simulink model "GVCU_HIL"  (R2026a)
settings: Solver=ode3  StartTime=0  StopTime=2474  FixedStep=0.0002
model workspace (MAT data in the model file):
  CANoelibParameters : object (value not decoded)
values from neighbouring files (symbols this model uses):
  acc_pedal_data = pedal_data.accelerator_pedal_position_t0    [Vehicle_Simulink_init.m]
  acc_pedal_time = pedal_data.t0    [Vehicle_Simulink_init.m]
  brk_pedal_data = brake_pedal_data.shared_brakes_drvrBrkPedlPerc_t0    [Vehicle_Simulink_init.m]
  brk_pedal_time = brake_pedal_data.t0    [Vehicle_Simulink_init.m]
  cycle_len = zeros(1, num_cycles)    [Vehicle_Simulink_init.m]
  cycle_speed_matrix = zeros(max_cycle_len, num_cycles)    [Vehicle_Simulink_init.m]
  cycle_time_matrix = zeros(max_cycle_len, num_cycles)    [Vehicle_Simulink_init.m]
  veh_speed_data = speed_data.shared_dynamicsVso_vehVelLgt_t0    [Vehicle_Simulink_init.m]
  veh_speed_time = speed_data.t0    [Vehicle_Simulink_init.m]
undefined symbols (not defined in the file or in its folder): Active, AuxActive, bat, environment, FL_prs_voltage, FR_prs_voltage, pos, RL_prs_voltage, RR_prs_voltage, tir, veh, VGetRawValueFlag, Voltage, VT2816_1_Ch1, VT2816_1_Ch2, VT2816_1_Ch3, VT2816_1_Ch4, VT2816_3_Ch13, VT2816_3_Ch14, VT7101_1_Out2, VT7820_2_Channel1, VT7820_2_Channel2, VT7820_2_Channel3, VT7820_2_Channel4, VTS
libraries: canoelib x144, autolibsharedcoupling x21, autolibcoupling x9, autolibshared x5, simulink_extras x4, simulink x4, slpidlib x3, autolibshareddiff x3, autolibutils x1, autolibdatasheetbattery x1, autolibmappedmotor x1, sl_discontinuities x1
(part 6 of 9)

== system GVCU_HIL/Powertrain (EV)/EM ==
  note: recuperation
  TrqCmd : Inport
  EMSpd : Inport  Port=2
  Bus Creator : BusCreator  Inputs=3
  Constant : Constant
  Constant1 : Constant  Value=-1
  Datasheet Battery2 : autolibdatasheetbattery/Datasheet Battery  CapacityCtrl=Parameter  OutputVlt=Unfiltered  BattChargeMax=14.118  Em=[706.554, 720.834, 735.216, 742.356, 750.72, 765.714, 790.704, 810.798, 832.524, 855.372]  SOCEmBp=[0.1, 0.2, 0.3, 0.4, 0.5, 0.6, 0.7, 0.8, 0.9, 1]  RInt=[0.14, 0.12;0.14, 0.12;0.14, 0.12;0.14, 0.12;0.14, 0.12;0.14, 0.12;0.155, 0.135;0.16, 0.145;0.165, 0.155;0.175, 0.175]'  BattTempBp=|  SOCRintBp=[0.1, 0.2, 0.3, 0.4, 0.5, 0.6, 0.7, 0.8, 0.9, 1]  Ns=1  Np=1  BattCapInit=14.118*bat.SoC_init  Tc=1/1000  Vinit=4.221  RefBlkName='autolibdatasheetbattery/Datasheet Battery'
      | [318.15,
      | 333.15
      | ]
  Mapped Motor : autolibmappedmotor/Mapped Motor  w_Tmax_bp_ext=w_Tmax_bp  Tmax_w_V_ext=Tmax_w_V  w_Tmin_bp_ext=w_Tmin_bp  Tmin_w_V_ext=Tmin_w_V  port_config=Speed  param_by=Tabulated torque-speed envelope  w_t=vEM  T_t=MEM  torque_max=.1  power_max=30  SpreadsheetTqLimitsFileName=MotorCalibrationImportData.xlsx  Tmax_w_V=[0.09 0.09 0.09;0.08 0.08 0.08;0.07 0.07 0.07;0 0 0]  w_Tmax_bp=[ 0 375 750 800 ]  V_Tmax_bp=[500 750 900]  Tmin_w_V=[-0.09 -0.09 -0.09;-0.08 -0.08 -0.08;-0.07 -0.07 -0.07;0 0 0]  w_Tmin_bp=[ 0 375 750 800 ]  V_Tmin_bp=[500 750 900]  Tc=0.02  param_loss=Tabulated loss data  SpreadsheetLossFileName=MotorCalibrationImportData.xlsx  SpreadsheetEffFileName=MotorCalibrationImportData.xlsx  eff=100  w_eff=375  T_eff=0.08  Piron=0  Pbase=0  w_eff_bp=eff_EM_speed  T_eff_bp=eff_EM_torque  Temp_eff_bp=[233.15 293.15 373.15]  V_eff_bp=[500 700 900]  losses_table=eff_EM_loss'  losses_table_3d=cat(3,[1.49 1.67 2.21 3.10; 0.42 0.69 1.14 2.03; 0.06 0.24 0.78 1.68; 0.42 0.69 1.14 2.03; 1.49 1.67 2.21 3.10],[1.49 1.67 2.21 3.10; 0.42 0.69 1.14 2.03; 0.06 0.24 0.78 1.68; 0.42 0.69 1.14 2.03; 1.49 1.67 2.21 3.10],[1.49 1.67 2.21 3.10; 0.42 0.69 1.14 2.03; 0.06 0.24 0.78 1.68; 0.42 0.69 1.14 2.03; 1.49 1.67 2.21 3.10])  losses_table_4d=cat(4,cat(3,[1.5645 0.441 0.063 0.441 1.5645;1.7535 0.7245 0.252 0.7245 1.7535;2.3205 1.197 0.819 1.197 2.3205;3.255 2.1315 1.764 2.1315 3.255],[1.5645 0.441 0.063 0.441 1.5645;1.7535 0.7245 0.252 0.7245 1.7535;2.3205 1.197 0.819 1.197 2.3205;3.255 2.1315 1.764 2.1315 3.255],[1.5645 0.441 0.063 0.441 1.5645;1.7535 0.7245 0.252 0.7245 1.7535;2.3205 1.197 0.819 1.197 2.3205;3.255 2.1315 1.764 2.1315 3.255]),cat(3,[1.49 0.42 0.06 0.42 1.49;1.67 0.69 0.24 0.69 1.67;2.21 1.14 0.78 1.14 2.21;3.1 2.03 1.68 2.03 3.1],[1.49 0.42 0.06 0.42 1.49;1.67 0.69 0.24 0.69 1.67;2.21 1.14 0.78 1.14 2.21;3.1 2.03 1.68 2.03 3.1],[1.49 0.42 0.06 0.42 1.49;1.67 0.69 0.24 0.69 1.67;2.21 1.14 0.78 1.14 2.21;3.1 2.03 1.68 2.03 3.1]),cat(3,[1.5347 0.4326 0.0618 0.4326 1.5347;1.7201 0.7107 0.2472 0.7107 1.7201;2.2763 1.1742 0.8034 1.1742 2.2763;3.193 2.0909 1.7304 2.0909 3.193],[1.5347 0.4326 0.0618 0.4326 1.5347;1.7201 0.7107 0.2472 0.7107 1.7201;2.2763 1.1742 0.8034 1.1742 2.2763;3.193 2.0909 1.7304 2.0909 3.193],[1.5347 0.4326 0.0618 0.4326 1.5347;1.7201 0.7107 0.2472 0.7107 1.7201;2.2763 1.1742 0.8034 1.1742 2.2763;3.193 2.0909 1.7304 2.0909 3.193]))  efficiency_table=[95 95 95 95; 95 95 95 95; 95 95 95 95; 95 95 95 95; 95 95 95 95]  efficiency_table_3d=cat(3,[95 95 95 95; 95 95 95 95; 95 95 95 95; 95 95 95 95; 95 95 95 95],[95 95 95 95; 95 95 95 95; 95 95 95 95; 95 95 95 95; 95 95 95 95],[95 95 95 95; 95 95 95 95; 95 95 95 95; 95 95 95 95; 95 95 95 95])  efficiency_table_4d=cat(4,cat(3,90*ones(5,4)',90*ones(5,4)',90*ones(5,4)'),cat(3,95*ones(5,4)',95*ones(5,4)',95*ones(5,4)'),cat(3,92*ones(5,4)',92*ones(5,4)',92*ones(5,4)'))  J=5e-6  b=1e-5  omega_o=0  T_t_extended=[591.1765761 597.3209021 603.5893235 609.9750859 616.4522479 623.0217147 629.6859649 636.4772464 643.4544242 650.5325557 657.7142528 665.0004238 672.3918517 679.8891731 687.4928554 695.2382707 703.2239794 711.3175267 719.5183987 727.8257293 736.2382506 744.7548459 753.4914197 762.3651559 771.3359703 780.40539 789.5706985 798.8284396 808.4176374 818.1172796 827.8944537 837.7411079 847.6338253 857.4187059 867.2137586 877.0119255 886.7904649 896.5231126 906.1796142 915.3256846 924.6270531 933.8736555 942.8047497 951.8719913 960.6156155 968.6277666 976.0298627 982.43675 988.6022535 994.0259096 997.4001374 999.7922394 1000.534965 1000.5472 1000.5472 1000.5472 1000.5472 1000.5472 1000.5472 1000.5472 1000.5472 1000.5472 1000.5472 1000.5472 1000.5472 1000.5472 1000.5472 1000.5472 1000.5472 1000.5472 1000.5472 1000.5472 1000.5472 1000.5472 1000.5472 1000.5472 1000.5472 1000.5472 1000.5472 1000.5472 1000.5472 1000.5472 1000.5472 1000.5472 1000.5472 1000.5472 1000.5472 1000.5472 1000.5472 1000.5472 1000.5472 1000.5472 1000.5472 1000.5472 1000.5472 1000.5472 1000.5472 1000.5472 1000.5472 1000.5472 1000.5472 1000.5472 1000.5472 1000.5472 1000.5472 1000.5472 1000.5472 1000.5472 1000.5472 1000.5472 1000.5472 1000.5472 1000.5472 1000.5472 1000.5472 1000.5472 1000.5472 1000.5472 1000.5472 1000.5472 1000.5472 1000.5472 1000.5472 1000.5472 1000.5472 1000.5472 1000.5472 1000.5472 1000.5472 1000.5472 1000.5472 1000.5472 1000.5472 1000.5472 1000.5472 1000.5472 1000.5472 1000.5472 1000.5472 1000.5472 1000.5472 1000.5472 1000.5472 1000.5472 1000.5472 1000.5472 1000.5472 1000.5472 1000.534965 999.7922394 997.4001374 994.0259096 988.6022535 982.43675 976.0298627 968.6277666 960.6156155 951.8719913 942.8047497 933.8736555 924.6270531 915.3256846 906.1796142 896.5231126 886.7904649 877.0119255 867.2137586 857.4187059 847.6338253 837.7411079 827.8944537 818.1172796 808.4176374 798.8284396 789.5706985 780.40539 771.3359703 762.3651559 753.4914197 744.7548459 736.2382506 727.8257293 719.5183987 711.3175267 703.2239794 695.2382707 687.4928554 679.8891731 672.3918517 665.0004238 657.7142528 650.5325557 643.4544242 636.4772464 629.6859649 623.0217147 616.4522479 609.9750859 603.5893235 597.3209021 591.1765761]  w_t_extended=[-1047.197551 -1036.725576 -1026.2536 -1015.781625 -1005.309649 -994.8376736 -984.3656981 -973.8937226 -963.4217471 -952.9497716 -942.4777961 -932.0058206 -921.5338451 -911.0618695 -900.589894 -890.1179185 -879.645943 -869.1739675 -858.701992 -848.2300165 -837.758041 -827.2860654 -816.8140899 -806.3421144 -795.8701389 -785.3981634 -774.9261879 -764.4542124 -753.9822369 -743.5102613 -733.0382858 -722.5663103 -712.0943348 -701.6223593 -691.1503838 -680.6784083 -670.2064328 -659.7344573 -649.2624817 -638.7905062 -628.3185307 -617.8465552 -607.3745797 -596.9026042 -586.4306287 -575.9586532 -565.4866776 -555.0147021 -544.5427266 -534.0707511 -523.5987756 -513.1268001 -502.6548246 -492.1828491 -481.7108736 -471.238898 -460.7669225 -450.294947 -439.8229715 -429.350996 -418.8790205 -408.407045 -397.9350695 -387.4630939 -376.9911184 -366.5191429 -356.0471674 -345.5751919 -335.1032164 -324.6312409 -314.1592654 -303.6872898 -293.2153143 -282.7433388 -272.2713633 -261.7993878 -251.3274123 -240.8554368 -230.3834613 -219.9114858 -209.4395102 -198.9675347 -188.4955592 -178.0235837 -167.5516082 -157.0796327 -146.6076572 -136.1356817 -125.6637061 -115.1917306 -104.7197551 -94.24777961 -83.7758041 -73.30382858 -62.83185307 -52.35987756 -41.88790205 -31.41592654 -20.94395102 -10.47197551 0 10.47197551 20.94395102 31.41592654 41.88790205 52.35987756 62.83185307 73.30382858 83.7758041 94.24777961 104.7197551 115.1917306 125.6637061 136.1356817 146.6076572 157.0796327 167.5516082 178.0235837 188.4955592 198.9675347 209.4395102 219.9114858 230.3834613 240.8554368 251.3274123 261.7993878 272.2713633 282.7433388 293.2153143 303.6872898 314.1592654 324.6312409 335.1032164 345.5751919 356.0471674 366.5191429 376.9911184 387.4630939 397.9350695 408.407045 418.8790205 429.350996 439.8229715 450.294947 460.7669225 471.238898 481.7108736 492.1828491 502.6548246 513.1268001 523.5987756 534.0707511 544.5427266 555.0147021 565.4866776 575.9586532 586.4306287 596.9026042 607.3745797 617.8465552 628.3185307 638.7905062 649.2624817 659.7344573 670.2064328 680.6784083 691.1503838 701.6223593 712.0943348 722.5663103 733.0382858 743.5102613 753.9822369 764.4542124 774.9261879 785.3981634 795.8701389 806.3421144 816.8140899 827.2860654 837.758041 848.2300165 858.701992 869.1739675 879.645943 890.1179185 900.589894 911.0618695 921.5338451 932.0058206 942.4777961 952.9497716 963.4217471 973.8937226 984.3656981 994.8376736 1005.309649 1015.781625 1026.2536 1036.725576 1047.197551]  KLossIron=0  KLossCopper=0  x_w_eff_vec=[-1151.91730631626 -1099.55742875643 -1047.1975511966 -994.837673636768 -942.477796076938 -890.117918517108 -837.758040957278 -785.398163397448 -733.038285837618 -680.678408277789 -628.318530717959 -575.958653158129 -523.598775598299 -471.238898038469 -418.879020478639 -366.519142918809 -314.159265358979 -261.799387799149 -209.43951023932 -157.07963267949 -104.71975511966 -52.3598775598299 0 52.3598775598299 104.71975511966 157.07963267949 209.43951023932 261.799387799149 314.159265358979 366.519142918809 418.879020478639 471.238898038469 523.598775598299 575.958653158129 628.318530717959 680.678408277789 733.038285837618 785.398163397448 837.758040957278 890.117918517108 942.477796076938 994.837673636768 1047.1975511966 1099.55742875643 1151.91730631626]  x_T_eff_vec=[-1100 -1000 -900 -800 -700 -600 -500 -400 -300 -200 -100 0 100 200 300 400 500 600 700 800 900 1000 1100]  x_tmp_eff_vec=[-0.09 -0.06 -0.03 0 0.03 0.06 0.09]  x_V_eff_vec=[500 700 900]  x_losses_mat=[216963.75801 216996.227265 206067.578848888 197642.105612969 153300.977107873 108080.0572 72647.49686 49091.12876 32858.35954 22129.50585 16054.65961 13895.5575 16054.65961 22129.50585 32858.35954 49091.12876 72647.49686 108080.0572 153300.977107873 197642.105612969 206067.578848888 216996.227265 216963.75801;231488.890349682 223059.669245745 204039.410989428 184347.436290099 134715.207987873 87903.07434 59579.3291 40088.01049 26456.98289 17357.92244 12141.80753 10371.65043 12141.80753 17357.92244 26456.98289 40088.01049 59579.3291 87903.07434 134715.207987873 184347.436290099 204039.410989428 223059.669245745 231488.890349682;189437.61777 184243.717645 168828.860886349 149567.396061484 106341.0793 71543.39502 48728.82856 32631.17131 21200.63415 13523.21842 9082.511039 7599.257015 9082.511039 13523.21842 21200.63415 32631.17131 48728.82856 71543.39502 106341.0793 149567.396061484 168828.860886349 184243.717645 189437.61777;192935.210247969 180472.732852227 158159.379341563 128824.526141484 85033.49473 58268.77005 39819.67343 26520.36346 16954.07308 10512.49572 6795.723221 5551.699791 6795.723221 10512.49572 16954.07308 26520.36346 39819.67343 58268.77005 85033.49473 128824.526141484 158159.379341563 180472.732852227 192935.210247969;155580.94976 146657.635255 128253.525153809 99653.02374 68484.12552 47553.88198 32618.55146 21582.78411 13649.90656 8283.638962 5179.539664 4137.799792 5179.539664 8283.638962 13649.90656 21582.78411 32618.55146 47553.88198 68484.12552 99653.02374 128253.525153809 146657.635255 155580.94976;129871.92913 122034.11486 105085.58551254 79050.02512 55595.93478 39058.96664 26875.37628 17810.73423 11257.11835 6780.923192 4207.530813 3337.757479 4207.530813 6780.923192 11257.11835 17810.73423 26875.37628 39058.96664 55595.93478 79050.02512 105085.58551254 122034.11486 129871.92913;121153.617618809 109771.61748004 89648.9827825395 64650.328115 45845.19165 32428.08909 22502.00533 15114.9243 9718.777596 5996.518981 3863.3287 3140.213628 3863.3287 5996.518981 9718.777596 15114.9243 22502.00533 32428.08909 45845.19165 64650.328115 89648.9827825395 109771.61748004 121153.617618809;102556.24812 91278.85608 71630.91 52385.27894 38216.08162 27475.52514 19481.57898 13474.37309 8882.641372 5572.115215 3606.515506 2926.128354 3606.515506 5572.115215 8882.641372 13474.37309 19481.57898 27475.52514 38216.08162 52385.27894 71630.91 91278.85608 102556.24812;92639.38668 78466.74469 58974.42114 44130.45585 32866.66791 24279.62179 17574.57444 12226.59488 8087.099664 5111.496599 3338.107135 2693.28051 3338.107135 5111.496599 8087.099664 12226.59488 17574.57444 24279.62179 32866.66791 44130.45585 58974.42114 78466.74469 92639.38668;79967.9231 65252.31828 50217.87648 38582.89904 29358.82442 21876.86476 15843.69216 11050.03907 7345.279935 4716.81461 3049.949208 2447.800925 3049.949208 4716.81461 7345.279935 11050.03907 15843.69216 21876.86476 29358.82442 38582.89904 50217.87648 65252.31828 79967.9231;71978.46712 56942.67707 44620.193540345 34536.29737 26359.17892 19662.58912 14256.71192 9978.264251 6676.859148 4212.93021 2749.898985 2203.255002 2749.898985 4212.93021 6676.859148 9978.264251 14256.71192 19662.58912 26359.17892 34536.29737 44620.193540345 56942.67707 71978.46712;64307.84812 50926.57919 39881.7876028249 30906.36917 23642.38009 17643.48449 12827.89413 8955.839244 5908.871417 3769.457125 2456.82187 1959.642739 2456.82187 3769.457125 5908.871417 8955.839244 12827.89413 17643.48449 23642.38009 30906.36917 39881.7876028249 50926.57919 64307.84812;57412.00559 45490.46778 35625.4624361057 27664.12726 21175.22168 15830.68178 11431.8958 7924.881587 5262.677959 3349.859461 2170.073056 1716.964138 2170.073056 3349.859461 5262.677959 7924.881587 11431.8958 15830.68178 21175.22168 27664.12726 35625.4624361057 45490.46778 57412.00559;51224.02114 40607.66616 31797.2898800987 24744.95924 18926.39057 14056.32423 10116.63964 7040.932836 4665.120485 2950.41808 1889.056344 1475.219198 1889.056344 2950.41808 4665.120485 7040.932836 ...(+8994 chars)]  x_losses_mat_3d=[37.8947368421052 25.2631578947368 12.6315789473684 0 12 24 36;18.9473684210526 12.6315789473684 6.3157894736842 0 5.99999999999999 12 18;0 0 0 0 0 0 0;18 12 5.99999999999999 0 6.3157894736842 12.6315789473684 18.9473684210526;36 24 12 0 12.6315789473684 25.2631578947368 37.8947368421052]  x_losses_mat_4d=cat(4,cat(3,[1.5645 0.441 0.063 0.441 1.5645;1.7535 0.7245 0.252 0.7245 1.7535;2.3205 1.197 0.819 1.197 2.3205;3.255 2.1315 1.764 2.1315 3.255],[1.5645 0.441 0.063 0.441 1.5645;1.7535 0.7245 0.252 0.7245 1.7535;2.3205 1.197 0.819 1.197 2.3205;3.255 2.1315 1.764 2.1315 3.255],[1.5645 0.441 0.063 0.441 1.5645;1.7535 0.7245 0.252 0.7245 1.7535;2.3205 1.197 0.819 1.197 2.3205;3.255 2.1315 1.764 2.1315 3.255]),cat(3,[1.49 0.42 0.06 0.42 1.49;1.67 0.69 0.24 0.69 1.67;2.21 1.14 0.78 1.14 2.21;3.1 2.03 1.68 2.03 3.1],[1.49 0.42 0.06 0.42 1.49;1.67 0.69 0.24 0.69 1.67;2.21 1.14 0.78 1.14 2.21;3.1 2.03 1.68 2.03 3.1],[1.49 0.42 0.06 0.42 1.49;1.67 0.69 0.24 0.69 1.67;2.21 1.14 0.78 1.14 2.21;3.1 2.03 1.68 2.03 3.1]),cat(3,[1.5347 0.4326 0.0618 0.4326 1.5347;1.7201 0.7107 0.2472 0.7107 1.7201;2.2763 1.1742 0.8034 1.1742 2.2763;3.193 2.0909 1.7304 2.0909 3.193],[1.5347 0.4326 0.0618 0.4326 1.5347;1.7201 0.7107 0.2472 0.7107 1.7201;2.2763 1.1742 0.8034 1.1742 2.2763;3.193 2.0909 1.7304 2.0909 3.193],[1.5347 0.4326 0.0618 0.4326 1.5347;1.7201 0.7107 0.2472 0.7107 1.7201;2.2763 1.1742 0.8034 1.1742 2.2763;3.193 2.0909 1.7304 2.0909 3.193]))  CalLossMapData={}  CalLossWithTempMapData={}  aMode=1  RefBlkName='autolibmappedmotor/Mapped Motor'
      settings: LibrarySourceBlock=autolibemachines/Mapped Motor
  Product : Product
  Product1 : Product
  Switch : Switch  SaturateOnIntegerOverflow=off  InputSameDT=off
  System Variable Output : canoelib/CANoe I//O/System Variable Output  Commented=on  nsName=Checker_Simulink  sysVarName=Test_param  arrayIndex=-1  rawValue=Default  dataType=Default  dataTypeDB=int32  hasEncoding=off  dataTypeCANoe=Get from CANoe
      settings: AttributesFormatString=%<nsName>::%<sysVarName>  SourceProductName=Vector CANoe
  Temperature1 : Constant  Value=320
  Terminator : Terminator
  Transfer Fcn : TransferFcn  Denominator=[0.001 1]
  Info : Outport
  EMTrq : Outport  Port=2  VectorParamsAs1DForOutWhenUnconnected=off
  tag scope: BatteryCurrent=global, BatteryVoltage=global
  wires:
  Mapped Motor/2 -> Transfer Fcn/1
  Transfer Fcn/1 -> Datasheet Battery2/1, [BatteryCurrent]
  Datasheet Battery2/1 -> [Battery]  "Battery"
  [EMSpd] -> Bus Creator/1  "EMSpd"
  [Battery] -> Bus Creator/3  "Battery"
  Datasheet Battery2/2 -> Mapped Motor/1, [BatteryVoltage]  "New"
  Temperature1/1 -> Datasheet Battery2/2
  Bus Creator/1 -> Info/1
  EMSpd/1 -> Mapped Motor/2, [EMSpd]  "EMSpd"
  Product1/1 -> EMTrq/1, Bus Creator/2  "EMTrq"
  Mapped Motor/1 -> Terminator/1
  Constant/1 -> Switch/1
  Constant1/1 -> Switch/3
  Switch/1 -> Product/2, System Variable Output/1, Product1/2  "1 or -1"
  Product/1 -> Mapped Motor/3
  Mapped Motor/3 -> Product1/1  "EMTrq"
  TrqCmd/1 -> Switch/2, Product/1  "TrqCmd"

== system GVCU_HIL/Powertrain (EV)/FWD_ELEC_Powertrain ==
  EMTrq : Inport
  Veh : Inport  Port=2
  Bus Selector : BusSelector  OutputSignals=Wheels.Omega
  Constant2 : Constant  Value=0
  Constant3 : Constant  Value=0
  Demux : Demux
  FL : autolibsharedcoupling/Torsional Compliance  port_config=Simulink  extInfo=off  k=5e4  b=4e2  theta_o=0  domega_o=0  omega_c=3000  blkID=0  aMode=1
  FL_Clutch : autolibcoupling/Disc Clutch  port_config=Simulink  Reff=.091/2  Ndisk=9  Aeff=0.006283185  Peng=320000  Jin=.1  Jout=.1  muk=.088  mus=.089  bin=.001  bout=.001  win_o=pos.xdot_0/veh.TyreLoadedRadius_F  wout_o=pos.xdot_0/veh.TyreLoadedRadius_F  tauC=1  InitiallyLocked=off  maxAbsSpd=3000  blkID=1
  FR : autolibsharedcoupling/Torsional Compliance  port_config=Simulink  extInfo=off  k=5e4  b=4e2  theta_o=0  domega_o=0  omega_c=3000  blkID=0  aMode=1
  FR_Clutch : autolibcoupling/Disc Clutch  port_config=Simulink  Reff=.091/2  Ndisk=9  Aeff=0.006283185  Peng=320000  Jin=.1  Jout=.1  muk=.088  mus=.089  bin=.001  bout=.001  win_o=pos.xdot_0/veh.TyreLoadedRadius_F  wout_o=pos.xdot_0/veh.TyreLoadedRadius_F  tauC=.01  InitiallyLocked=off  maxAbsSpd=3000  blkID=1
  From1 : From  Commented=on  GotoTag=FR_prs  TagVisibility=global
  Gain : Gain  Gain=1/2.71
  Gain1 : Gain  Gain=1/2.71
  Gain2 : Gain  Gain=30/pi
  Mux1 : Mux
  Rotational Inertia : autolibsharedcoupling/Rotational Inertia  port_config=Simulink  extInfo=off  externJ=off  J=.1  b=.001  omega_o=0  blkID=0  aMode=1
      settings: LibrarySourceBlock=autolibcoupling/Rotational Inertia
  Split Torsional Compliance : autolibsharedcoupling/Split Torsional Compliance  port_config=Simulink  cplrMode=Shaft split  extInfo=off  k1=5e4  b1=4e2  omega1_c=1000  theta1_o=0  domega1_o=0  k2=5e4  b2=4e2  omega2_c=1000  theta2_o=0  domega2_o=0  blkID=0  aMode=1
      settings: LibrarySourceBlock=autolibcoupling/Split Torsional Compliance
  Terminator{,1..3} (4 alike) : Terminator
  EM_Spd : Outport
  Axl_Trq1 : Outport  Port=2
  tag scope: Axl_front_Spd=global, Split_tors_FL=global, Split_tors_FR=global
  wires:
  Constant3/1 -> Mux1/4
  Constant2/1 -> Mux1/3
  Mux1/1 -> Axl_Trq1/1
  FR/2 -> Mux1/2  "T_FR"
  FL/2 -> Mux1/1  "T_FL"
  EMTrq/1 -> Rotational Inertia/1
  Split Torsional Compliance/1 -> Gain1/1
  Demux/1 -> FL/2
  Split Torsional Compliance/3 -> [Split_tors_FR], FR_Clutch/2  "Front_right_clutch"
  FL_Clutch/1 -> Terminator3/1
  [FL_prs] -> FR_Clutch/1, FL_Clutch/1
  Veh/1 -> Bus Selector/1
  FR_Clutch/2 -> Split Torsional Compliance/3
  FR/1 -> FR_Clutch/3
  Split Torsional Compliance/2 -> [Split_tors_FL], FL_Clutch/2  "Front_left_clutch"
  Rotational Inertia/1 -> EM_Spd/1, Gain/1
  Gain/1 -> Gain2/1, Split Torsional Compliance/1
  Bus Selector/1 -> Demux/1  "<Omega>"
  FR_Clutch/3 -> FR/1
  Demux/4 -> Terminator1/1
  FR_Clutch/1 -> Terminator2/1
  FL_Clutch/2 -> Split Torsional Compliance/2
  Demux/2 -> FR/2
  Demux/3 -> Terminator/1
  FL_Clutch/3 -> FL/1
  FL/1 -> FL_Clutch/3
  Gain1/1 -> Rotational Inertia/2
  Gain2/1 -> [Axl_front_Spd]  "rpm"

== system GVCU_HIL/Powertrain (EV)/FWD_ELEC_Powertrain_sorted ==
  note: Front Bevel Ration
  EMTrq : Inport
  Veh : Inport  Port=2
  Bus Selector : BusSelector  OutputSignals=Wheels.Omega
  Constant2 : Constant  Value=0
  Constant3 : Constant  Value=0
  Demux : Demux
  FL : autolibsharedcoupling/Torsional Compliance  port_config=Simulink  extInfo=off  k=5e4  b=4e2  theta_o=0  domega_o=0  omega_c=3000  blkID=0  aMode=1
  FL_Clutch : autolibcoupling/Disc Clutch  port_config=Simulink  Reff=.091/2  Ndisk=9  Aeff=0.006283185  Peng=110000  Jin=.1  Jout=.1  muk=.088  mus=.089  bin=.001  bout=.001  win_o=pos.xdot_0/veh.TyreLoadedRadius_F  wout_o=pos.xdot_0/veh.TyreLoadedRadius_F  tauC=1  InitiallyLocked=off  maxAbsSpd=3000  blkID=1
  FR : autolibsharedcoupling/Torsional Compliance  port_config=Simulink  extInfo=off  k=5e4  b=4e2  theta_o=0  domega_o=0  omega_c=3000  blkID=0  aMode=1
  FR_Clutch : autolibcoupling/Disc Clutch  port_config=Simulink  Reff=.091/2  Ndisk=9  Aeff=0.006283185  Peng=110000  Jin=.1  Jout=.1  muk=.088  mus=.089  bin=.001  bout=.001  win_o=pos.xdot_0/veh.TyreLoadedRadius_F  wout_o=pos.xdot_0/veh.TyreLoadedRadius_F  tauC=.01  InitiallyLocked=off  maxAbsSpd=3000  blkID=1
  Gain : Gain  Gain=1/2.71
  Gain1 : Gain  Gain=1/2.71
  Gain2 : Gain  Gain=30/pi
  Mux1 : Mux
  Rotational Inertia : autolibsharedcoupling/Rotational Inertia  port_config=Simulink  extInfo=off  externJ=off  J=.1  b=.001  omega_o=0  blkID=0  aMode=1
      settings: LibrarySourceBlock=autolibcoupling/Rotational Inertia
  Split Torsional Compliance : autolibsharedcoupling/Split Torsional Compliance  port_config=Simulink  cplrMode=Shaft split  extInfo=off  k1=5e4  b1=4e2  omega1_c=1000  theta1_o=0  domega1_o=0  k2=5e4  b2=4e2  omega2_c=1000  theta2_o=0  domega2_o=0  blkID=0  aMode=1
      settings: LibrarySourceBlock=autolibcoupling/Split Torsional Compliance
  Terminator{,1..3} (4 alike) : Terminator
  EM_Spd : Outport
  Axl_Trq1 : Outport  Port=2
  tag scope: Axl_front_Spd=global, Split_tors_FL=global, Split_tors_FR=global, T_FL=global, T_FR=global
  wires:
  Constant3/1 -> Mux1/4
  Constant2/1 -> Mux1/3
  Mux1/1 -> Axl_Trq1/1
  FR/2 -> [T_FR]  "T_FR"
  FL/2 -> [T_FL]  "T_FL"
  EMTrq/1 -> Rotational Inertia/1
  Split Torsional Compliance/1 -> Gain1/1
  Demux/1 -> FL/2
  Split Torsional Compliance/2 -> [Split_tors_FR], FR_Clutch/2  "Front_right_clutch"
  FL_Clutch/1 -> Terminator3/1
  [FR_prs] -> FR_Clutch/1
  Veh/1 -> Bus Selector/1
  FR_Clutch/2 -> Split Torsional Compliance/2
  FR/1 -> FR_Clutch/3
  Split Torsional Compliance/3 -> [Split_tors_FL], FL_Clutch/2  "Front_left_clutch"
  Rotational Inertia/1 -> EM_Spd/1, Gain/1
  Gain/1 -> Gain2/1, Split Torsional Compliance/1
  Bus Selector/1 -> Demux/1  "<Omega>"
  FR_Clutch/3 -> FR/1
  Demux/4 -> Terminator1/1
  FR_Clutch/1 -> Terminator2/1
  FL_Clutch/2 -> Split Torsional Compliance/3
  Demux/2 -> FR/2
  Demux/3 -> Terminator/1
  FL_Clutch/3 -> FL/1
  FL/1 -> FL_Clutch/3
  Gain1/1 -> Rotational Inertia/2
  Gain2/1 -> [Axl_front_Spd]  "rpm"
  [T_FR] -> Mux1/2
  [T_FL] -> Mux1/1
  [FL_prs] -> FL_Clutch/1

== system GVCU_HIL/Powertrain (EV)/PID Speed Controller ==
  note: feed forward value
  speed_feedback : Inport
  trq_lim : Inport  Port=2
  speed_req : Inport  Port=3
  trq_req : Inport  Port=4
  reset : Inport  Port=5
  Add : Sum
  Add1 : Sum
  Clock : Clock
  Constant : Constant  Commented=on  Value=0
  Gain : Gain  Gain=-1
  MATLAB Function : MATLAB Function  TreatAsAtomicUnit=on
  PID Controller1 : slpidlib/PID Controller  Controller=PI  Form=Parallel  TimeDomain=Discrete-time  UseExternalTs=off  SampleTime=0.0004  IntegratorMethod=Trapezoidal  FilterMethod=Forward Euler  ControllerParametersSource=internal  P=0.78  I=0.01  UseKiTs=off  D=0  UseExternalDerivativeSource=off  N=100  UseFilter=on  TunerSelectOption=Transfer Function Based (PID Tuner App)  InitialConditionSource=internal  InitialConditionForIntegrator=0  InitialConditionForFilter=0  DifferentiatorICPrevScaledInput=0  ExternalReset=level  TrackingMode=off  Kt=1  LimitOutput=on  SatLimitsSource=internal  UpperSaturationLimit=1000  LowerSaturationLimit=-1000  LinearizeAsGain=on  AntiWindupMode=back-calculation  Kb=0.005  LimitIntegrator=on  UpperIntegratorSaturationLimit=inf  LowerIntegratorSaturationLimit=-inf  POutMin=[]  POutMax=[]  IOutMin=[]  IOutMax=[]  DOutMin=[]  DOutMax=[]  NOutMin=[]  NOutMax=[]  SumOutMin=[]  SumOutMax=[]  SaturationOutMin=[]  SaturationOutMax=[]  PParamMin=[]  PParamMax=[]  IParamMin=[]  IParamMax=[]  DParamMin=[]  DParamMax=[]  NParamMin=[]  NParamMax=[]  KbParamMin=[]  KbParamMax=[]  KtParamMin=[]  KtParamMax=[]  KbOutMin=[]  KbOutMax=[]  KtOutMin=[]  KtOutMax=[]  IntegratorOutMin=[]  IntegratorOutMax=[]  FilterOutMin=[]  FilterOutMax=[]  SumI1OutMin=[]  SumI1OutMax=[]  SumI2OutMin=[]  SumI2OutMax=[]  SumI3OutMin=[]  SumI3OutMax=[]  SumI4OutMin=[]  SumI4OutMax=[]  SumDOutMin=[]  SumDOutMax=[]  DifferentiatorOutMin=[]  DifferentiatorOutMax=[]  FilterDiffOutCoefMin=[]  FilterDiffOutCoefMax=[]  ReciprocalOutMin=[]  ReciprocalOutMax=[]  SumDenOutMin=[]  SumDenOutMax=[]  SumNumOutMin=[]  SumNumOutMax=[]  DivideOutMin=[]  DivideOutMax=[]  UdiffTsProdOutMin=[]  UdiffTsProdOutMax=[]  NTsProdOutMin=[]  NTsProdOutMax=[]  UintegralTsProdOutMin=[]  UintegralTsProdOutMax=[]  UngainTsProdOutMin=[]  UngainTsProdOutMax=[]  ClampingZeroOutDataTypeStr=Inherit: Inherit via back propagation  ClampingZeroOutMin=[]  ClampingZeroOutMax=[]  FilterDenConstantOutDataTypeStr=Inherit: Inherit via back propagation  FilterDenConstantOutMin=[]  FilterDenConstantOutMax=[]  PCopyOutDataTypeStr=Inherit: Inherit via back propagation  PCopyOutMin=[]  PCopyOutMax=[]  NCopyOutDataTypeStr=Inherit: Inherit via back propagation  NCopyOutMin=[]  NCopyOutMax=[]  IntegratorContinuousStateAttributes=''  IntegratorStateMustResolveToSignalObject=off  IntegratorRTWStateStorageClass=Auto  FilterContinuousStateAttributes=''  FilterStateMustResolveToSignalObject=off  FilterRTWStateStorageClass=Auto  ParallelPVariant=InternalParameters  IdealPVariant=Disabled  IVariant=InternalParameters  DVariant=Disabled  IntegratorVariant=Discrete  SatVariant=Enabled  AWVariant=BackCalculation  PCopyVariant=Disabled  TRVariant=Disabled  FdbkBlocksVariant=Feedback  IdealPFdbkVariant=Passthrough  SatFdbkVariant=Enabled  DerivativeFilterVariant=Disabled  NVariant=Disabled  NCopyVariant=Disabled_SignalSpec  FilterICVariant=Disabled  IntegratorICVariant=InternalICs  ExternalResetVariant=ExternalReset  TRSumVariant=Passthrough  SumFdbkVariant=Enabled  SumVariant=Sum_PI  TsampFilterVariant=InternalTs  TsampNgainVariant=Passthrough  TsampIntegralVariant=Disabled_SignalSpec  ExternalSaturationOutDataTypeStr=Inherit: Same as second input  DerivativeSourceVariant=Disabled  PreIntVariant=InternalPreInt
  Saturation Dynamic : sl_discontinuities/Saturation Dynamic  OutMin=[]  OutMax=[]  OutDataTypeStr=Inherit: Same as second input  OutDataType=fixdt(1, 16)  OutScaling=2^-10  DoSatur=off
      settings: LibrarySourceBlock=|
      | simulink/Discontinuities/Saturation
      | Dynamic
  Subtract1 : Sum  Inputs=+-
  PID_EM_error : Outport
  Trq_cmd_elecMot : Outport  Port=2
  wires:
  speed_req/1 -> MATLAB Function/2(speed_req), Subtract1/1  "rad/s"
  MATLAB Function/1(reset_out) -> Add/1
  Clock/1 -> MATLAB Function/3(t)
  Saturation Dynamic/1 -> Add1/1
  Gain/1 -> Saturation Dynamic/3
  Subtract1/1 -> PID_EM_error/1, PID Controller1/1  "rpm"
  speed_feedback/1 -> Subtract1/2, MATLAB Function/1(EM_Spd)  "rad/s"
  PID Controller1/1 -> Saturation Dynamic/2
  Add1/1 -> Trq_cmd_elecMot/1
  trq_lim/1 -> Gain/1, Saturation Dynamic/1
  trq_req/1 -> Add1/2
  Add/1 -> PID Controller1/2
  reset/1 -> Add/2

== system GVCU_HIL/Powertrain (EV)/PID Speed Ctrl Mode ==
  note: 50 rpm / 500 us = 10472 rad/s /s
  speed_req : Inport
  speed_feedback : Inport  Port=2
  trq_req : Inport  Port=3
  trq_act : Inport  Port=4
  Action Port : ActionPort
  Clock : Clock
  Constant : Constant  Commented=on  Value=0
  Gain : Gain  Gain=-1
  MATLAB Function : MATLAB Function  TreatAsAtomicUnit=on
  MATLAB Function1 : MATLAB Function  TreatAsAtomicUnit=on
  Rate Limiter : RateLimiter  RisingSlewLimit=10472  FallingSlewLimit=-10472  SampleTimeMode=inherited
  Subtract1 : Sum  Inputs=+-
  Switch3 : Switch  Commented=on  Criteria=u2 > Threshold  SaturateOnIntegerOverflow=off  InputSameDT=off
  System Variable Input : canoelib/CANoe I//O/System Variable Input  Commented=on  nsName=Checker_Simulink  sysVarName=Panel_brake_pedal_perc  arrayIndex=-1  editSampleTime=0  rawValue=Default  dataType=Default  dataTypeDB=int32  hasEncoding=off  dataTypeCANoe=Get from CANoe
      settings: AttributesFormatString=%<nsName>::%<sysVarName>  SourceProductName=Vector CANoe
  Trq_cmd_elecMot : Outport
  PID_EM_error : Outport  Port=2
  wires:
  speed_req/1 -> Rate Limiter/1  "rad/s"
  trq_req/1 -> MATLAB Function1/2(trq_fwd)
  Subtract1/1 -> MATLAB Function1/1(spdErr_rads), PID_EM_error/1
  speed_feedback/1 -> MATLAB Function/1(EM_Spd), Subtract1/2  "rad/s"
  Clock/1 -> MATLAB Function/3(t)
  Rate Limiter/1 -> MATLAB Function/2(speed_req), Subtract1/1
  trq_act/1 -> MATLAB Function1/3(trq_act)
  Gain/1 -> MATLAB Function1/5(lim_neg)
  MATLAB Function1/1(trq_cmd) -> Trq_cmd_elecMot/1
  MATLAB Function/1(reset_out) -> MATLAB Function1/6(reset)
  Constant/1 -> Switch3/1
  System Variable Input/1 -> Switch3/2
  [Trq_limit_dyn] -> Gain/1, MATLAB Function1/4(lim_pos)

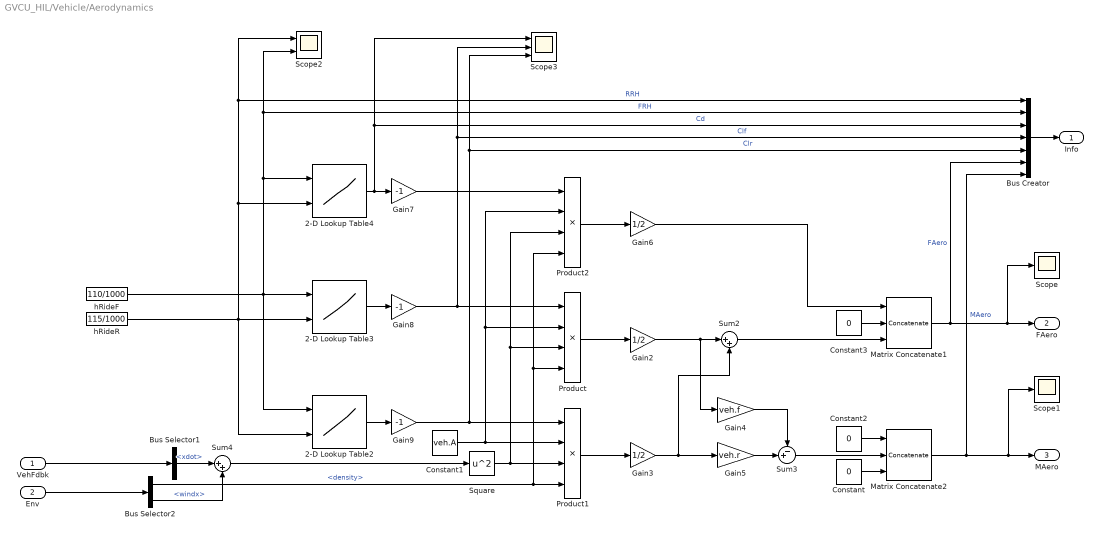
== system GVCU_HIL/Vehicle/Aerodynamics ==
  VehFdbk : Inport
  Env : Inport  Port=2
  2-D Lookup Table2 : Lookup_n-D  BreakpointsForDimension1=veh.aero.FRH  BreakpointsForDimension2=veh.aero.RRH  Table=veh.aero.Clr'  ExtrapMethod=Clip  UseLastTableValue=on  InternalRulePriority=Speed  RndMeth=Simplest
      settings: InputPortMap=u0,u1
  2-D Lookup Table3 : Lookup_n-D  BreakpointsForDimension1=veh.aero.FRH  BreakpointsForDimension2=veh.aero.RRH  Table=veh.aero.Clf'  ExtrapMethod=Clip  UseLastTableValue=on  InternalRulePriority=Speed  RndMeth=Simplest
      settings: InputPortMap=u0,u1
  2-D Lookup Table4 : Lookup_n-D  BreakpointsForDimension1=veh.aero.FRH  BreakpointsForDimension2=veh.aero.RRH  Table=veh.aero.Cd'  ExtrapMethod=Clip  UseLastTableValue=on  InternalRulePriority=Speed  RndMeth=Simplest
      settings: InputPortMap=u0,u1
  Bus Creator : BusCreator  Inputs=7
  Bus Selector1 : BusSelector  OutputSignals=BdyFrm.Cg.Vel.xdot
  Bus Selector2 : BusSelector  OutputSignals=Air.density,Wind.windx
  Constant : Constant  Value=0
  Constant1 : Constant  Value=veh.A
  Constant2 : Constant  Value=0
  Constant3 : Constant  Value=0
  Gain2 : Gain  Gain=1/2
  Gain3 : Gain  Gain=1/2
  Gain4 : Gain  Gain=veh.f
  Gain5 : Gain  Gain=veh.r
  Gain6 : Gain  Gain=1/2
  Gain7 : Gain  Gain=-1
  Gain8 : Gain  Gain=-1
  Gain9 : Gain  Gain=-1
  Matrix Concatenate1 : Concatenate  NumInputs=3  ConcatenateDimension=2
  Matrix Concatenate2 : Concatenate  NumInputs=3  ConcatenateDimension=2
  Product : Product  Inputs=4
  Product1 : Product  Inputs=4
  Product2 : Product  Inputs=4
  Scope : Scope
      settings: ActiveDisplayYMinimum=-135.81832  ActiveDisplayYMaximum=38.45391  DataLoggingVariableName=ScopeData2
  Scope1 : Scope
      settings: ActiveDisplayYMinimum=-4036.32096  ActiveDisplayYMaximum=448.48011
  Scope2 : Scope  NumInputPorts=2
      settings: ActiveDisplayYMinimum=-0.10098  ActiveDisplayYMaximum=0.2604
  Scope3 : Scope  NumInputPorts=3
      settings: ActiveDisplayYMinimum=-0.14892  ActiveDisplayYMaximum=0.36736  DataLoggingVariableName=ScopeData12
  Square : Math  Operator=square
  Sum2 : Sum  Inputs=|++
  Sum3 : Sum  Inputs=-+|
  Sum4 : Sum  Inputs=|++
  hRideF : Constant  Value=110/1000
  hRideR : Constant  Value=115/1000
  Info : Outport
  FAero : Outport  Port=2
  MAero : Outport  Port=3
  wires:
  Bus Creator/1 -> Info/1
  Matrix Concatenate2/1 -> MAero/1, Scope1/1, Bus Creator/7  "MAero"
  hRideF/1 -> 2-D Lookup Table3/1, 2-D Lookup Table2/1, 2-D Lookup Table4/1, Bus Creator/2, Scope2/2  "FRH"
  hRideR/1 -> 2-D Lookup Table4/2, Scope2/1, Bus Creator/1, 2-D Lookup Table3/2, 2-D Lookup Table2/2  "RRH"
  VehFdbk/1 -> Bus Selector1/1
  Sum4/1 -> Square/1
  Product/1 -> Gain2/1
  Product1/1 -> Gain3/1
  2-D Lookup Table3/1 -> Gain8/1
  Constant1/1 -> Product1/2, Product2/2, Product/2
  Gain2/1 -> Gain4/1, Sum2/1
  Sum2/1 -> Matrix Concatenate1/3
  Constant3/1 -> Matrix Concatenate1/2
  Matrix Concatenate1/1 -> Scope/1, FAero/1, Bus Creator/6  "FAero"
  Gain3/1 -> Gain5/1, Sum2/2
  Gain4/1 -> Sum3/1
  Gain5/1 -> Sum3/2
  Sum3/1 -> Matrix Concatenate2/2
  2-D Lookup Table4/1 -> Bus Creator/3, Scope3/1, Gain7/1  "Cd"
  Square/1 -> Product1/3, Product/3, Product2/3
  Product2/1 -> Gain6/1
  Gain6/1 -> Matrix Concatenate1/1
  Env/1 -> Bus Selector2/1
  Bus Selector2/1 -> Product2/4, Product/4, Product1/4  "<density>"
  Bus Selector2/2 -> Sum4/2  "<windx>"
  Bus Selector1/1 -> Sum4/1  "<xdot>"
  Constant2/1 -> Matrix Concatenate2/1
  Constant/1 -> Matrix Concatenate2/3
  2-D Lookup Table2/1 -> Gain9/1
  Gain7/1 -> Product2/1
  Gain8/1 -> Bus Creator/4, Scope3/2, Product/1  "Clf"
  Gain9/1 -> Bus Creator/5, Scope3/3, Product1/1  "Clr"

== system GVCU_HIL/Vehicle/Subsystem ==
  Cmd : Inport
  Bus Creator : BusCreator  Inputs=4
  Bus Creator1 : BusCreator  Inputs=1
  Bus Selector : BusSelector  OutputSignals=DecelCmd
  Constant : Constant
  Constant1 : Constant
  Demux : Demux
  Gain : Gain  Gain=100000
  Mux : Mux
  Product : Product
  Cntrl : Outport
  wires:
  Bus Creator1/1 -> Cntrl/1
  Demux/3 -> Bus Creator/3  "BrkPrsRL"
  Product/1 -> Gain/1  "bar"
  Demux/4 -> Bus Creator/4  "BrkPrsRR"
  Demux/1 -> Bus Creator/1  "BrkPrsFL"
  Gain/1 -> Demux/1  "Pa"
  Bus Selector/1 -> Product/2  "<DecelCmd>"
  Constant/1 -> Mux/2, Mux/1
  Cmd/1 -> Bus Selector/1
  Demux/2 -> Bus Creator/2  "BrkPrsFR"
  Mux/1 -> Product/1
  Bus Creator/1 -> Bus Creator1/1  "BrkPrs"
  Constant1/1 -> Mux/3, Mux/4

== system GVCU_HIL/Vehicle/Subsystem1 ==
  Cmd : Inport
  Bus Creator : BusCreator  Inputs=4
  Bus Creator1 : BusCreator  Inputs=1
  Bus Selector : BusSelector  OutputSignals=DecelCmd
  Constant : Constant
  Constant1 : Constant
  Constant2 : Constant  Value=veh.brake.brakeprs_gain
  Demux : Demux
  Gain : Gain  Gain=1/100
  Mux : Mux
  Product : Product
  Product1 : Product
  Cntrl : Outport
  wires:
  Bus Creator1/1 -> Cntrl/1
  Demux/3 -> Bus Creator/3  "BrkPrsRL"
  Product/1 -> Product1/2
  Demux/4 -> Bus Creator/4  "BrkPrsRR"
  Demux/1 -> Bus Creator/1  "BrkPrsFL"
  Product1/1 -> Demux/1
  Bus Selector/1 -> Gain/1  "<DecelCmd>"
  Constant/1 -> Mux/2, Mux/1
  Constant2/1 -> Product1/1
  Cmd/1 -> Bus Selector/1
  Demux/2 -> Bus Creator/2  "BrkPrsFR"
  Mux/1 -> Product/1
  Bus Creator/1 -> Bus Creator1/1  "BrkPrs"
  Constant1/1 -> Mux/3, Mux/4
  Gain/1 -> Product/2
